simulink model "Sim_sixDOF"  (R2023a)
settings: Solver=ode4  StartTime=0.0  StopTime=100  FixedStep=0.1  RelTol=1e-3
values from neighbouring files (symbols this model uses):
  a0_s2 = 0    [computeAeroForces.m]
  a0_s3 = 0    [computeAeroForces.m]
  a0_s4 = 0.05    [computeAeroForces.m]
  a0_s5 = 0.05    [computeAeroForces.m]
  AR_s2 = b_s2/c_s2    [computeSurfacePos.m]
  AR_s3 = b_s3/c_s3    [computeSurfacePos.m]
  AR_s4 = (b_s4 + b_s5)/c_s4    [computeSurfacePos.m]
  AR_s5 = (b_s4 + b_s5)/c_s5    [computeSurfacePos.m]
  area_s2 = c_s2 * b_s2    [computeSurfacePos.m]
  area_s3 = c_s3 * b_s3    [computeSurfacePos.m]
  area_s4 = c_s4 * b_s4    [computeSurfacePos.m]
  area_s5 = c_s5 * b_s5    [computeSurfacePos.m]
  c_s2 = componentMassesAndGeom(3,2)    [computeSurfacePos.m]
  c_s3 = componentMassesAndGeom(4,2)    [computeSurfacePos.m]
  c_s4 = componentMassesAndGeom(1,2)    [computeSurfacePos.m]
  c_s5 = componentMassesAndGeom(2,2)    [computeSurfacePos.m]
  CD0_s2 = 0.01    [computeAeroForces.m]
  CD0_s3 = 0.01    [computeAeroForces.m]
  CD0_s4 = 0.01    [computeAeroForces.m]
  CD0_s5 = 0.01    [computeAeroForces.m]
  CDa_s2 = 1    [computeAeroForces.m]
  CDa_s3 = 1    [computeAeroForces.m]
  CDa_s4 = 1    [computeAeroForces.m]
  CDa_s5 = 1    [computeAeroForces.m]
  CL0_s2 = 0    [computeAeroForces.m]
  CL0_s3 = 0    [computeAeroForces.m]
  CL0_s4 = 0.05    [computeAeroForces.m]
  CL0_s5 = 0.05    [computeAeroForces.m]
  CM0_s2 = 0    [computeAeroForces.m]
  CM0_s3 = 0    [computeAeroForces.m]
  CM0_s4 = -0.05    [computeAeroForces.m]
  CM0_s5 = -0.05    [computeAeroForces.m]
  CMa_s2 = 0    [computeAeroForces.m]
  CMa_s3 = 0    [computeAeroForces.m]
  CMa_s4 = 0    [computeAeroForces.m]
  CMa_s5 = 0    [computeAeroForces.m]
  e_s2 = 0.8    [computeAeroForces.m]
  e_s3 = 0.8    [computeAeroForces.m]
  e_s4 = 0.9    [computeAeroForces.m]
  e_s5 = 0.9    [computeAeroForces.m]
  elevator_sA = 0.435    [Sim_sixDOFdriverScript.m]
  i_s2 = 0    [computeAeroForces.m]
  i_s3 = 0    [computeAeroForces.m]
  i_s4 = 0.05    [computeAeroForces.m]
  i_s5 = 0.05    [computeAeroForces.m]
  Jxx = 1    [Sim_sixDOFdriverScript.m]
  Jxy = 0.    (= 0)    [Sim_sixDOFdriverScript.m]
  Jxz = 3    [Sim_sixDOFdriverScript.m]
  Jyx = 2    [Sim_sixDOFdriverScript.m]
  Jyy = 2    [Sim_sixDOFdriverScript.m]
  Jyz = 0    [Sim_sixDOFdriverScript.m]
  Jzx = Jxz    (= 3)    [Sim_sixDOFdriverScript.m]
  Jzy = Jyz    (= 0)    [Sim_sixDOFdriverScript.m]
  Jzz = 2    [Sim_sixDOFdriverScript.m]
  leftaileron_sA = 0.192/2    (= 0.096)    [Sim_sixDOFdriverScript.m]
  LL = 0.8    [Sim_sixDOFdriverScript.m]
  mixMatrixInv = inv(mixMatrix)    [Sim_sixDOFdriverScript.m]
  MM = 0.8    [Sim_sixDOFdriverScript.m]
  n_s2 = [0; 0; -1]    [computeAeroForces.m]
  n_s3 = [0; 1; 0]    [computeAeroForces.m]
  n_s4 = [0; 0; -1]    [computeAeroForces.m]
  n_s5 = [0; 0; -1]    [computeAeroForces.m]
  NN = 0.8    [Sim_sixDOFdriverScript.m]
  rEarth = 6378100    [Sim_sixDOFdriverScript.m]
  rightaileron_sA = 0.192/2    (= 0.096)    [Sim_sixDOFdriverScript.m]
  ro = 1.225    [computeAeroForces.m]
  rudder_sA = 0.0333    [Sim_sixDOFdriverScript.m]
  totMass = sum(componentMassesAndGeom(:,1))    [computeMassProps.m]
  x_S2_B_B = (x_S2_B_B_nominal + [0.25*c_s2 0 0]') - x_cg    [computeMassProps.m]
  x_S3_B_B = (x_S3_B_B_nominal + [0.25*c_s3 0 0]') - x_cg    [computeMassProps.m]
  x_S4_B_B = (x_S4_B_B_nominal + [0.25*c_s4 0 0]') - x_cg    [computeMassProps.m]
  x_S5_B_B = (x_S5_B_B_nominal + [0.25*c_s5 0 0]') - x_cg    [computeMassProps.m]
libraries: aerolibutil x3, simulink_extras x3, matrix_library x2, sharedtransform x2, simulink x2, sharedutil x1, vrlib x1
(part 2 of 2)

== matlab function Sim_sixDOF/Equations of Motion/Aero Forces and Moments/F&M Right Wing and Servo Surface (S5)/F&M in Body/Force Due to Lift and Drag ==
  data: lift input; forceLiftDragS5_B output; drag input; v_B_A_B input; n_s5 input
function forceLiftDragS5_B = fcn(lift, drag, v_B_A_B, n_s5)

forceLiftDrag_w = lift*n_s5 - [drag; 0; 0];
alpha = atan2(v_B_A_B(3), v_B_A_B(1));
beta = asin(v_B_A_B(2) / norm(v_B_A_B));

c_S_B = [cos(alpha), 0, sin(alpha); 0, 1, 0; -sin(alpha), 0, cos(alpha)] ;
c_W_S = [cos(beta), sin(beta), 0; -sin(beta), cos(beta), 0; 0,0,1];
c_W_B = c_W_S * c_S_B;

forceLiftDragS5_B = c_W_B' * forceLiftDrag_w;

== matlab function Sim_sixDOF/Equations of Motion/Aero Forces and Moments/F&M Right Wing and Servo Surface (S5)/F&M in Body/Moment S5 ==
  data: momSurf input; momS5_B output; FliftdragS input; n_s5 input; x_S5_B_B input
function momS5_B = fcn(momSurf, FliftdragS, n_s5, x_S5_B_B)
% Compute the moment at the respective surface
crot = [0,0,0; 0,0,-1; 0,1,0];

momS5_B = momSurf * crot* n_s5 + (cross(x_S5_B_B, FliftdragS));

== matlab function Sim_sixDOF/Equations of Motion/TransKin_RotKin_TansDynam/Rotational Kinematics_Quaternions/NormalizeQuaternion ==
  data: qin input; qoutNorm output
function qoutNorm = NormalizeQuaternion(qin)
qinMag = norm(qin);
qoutNorm = qin/qinMag;

== matlab function Sim_sixDOF/Equations of Motion/Aero Forces and Moments/F&M Horiz Stab Surface (S2)/F&M in Body/Moment S2 ==
  data: momSurf input; momS2_B output; FliftdragS input; n_s2 input; x_S2_B_B input
function momS2_B = fcn(momSurf, FliftdragS, n_s2, x_S2_B_B)
% Compute the moment at the respective surface
crot = [0,0,0; 0,0,-1; 0,1,0];

momS2_B = momSurf * crot* n_s2 + (cross(x_S2_B_B, FliftdragS));

== matlab function Sim_sixDOF/Equations of Motion/TransKin_RotKin_TansDynam/Rotational Kinematics_Quaternions/quaternionMultiplication ==
  data: q1 input; qResult output; q2 input
function qResult = quaternionMultiplication(q1,q2)
q1imag = [q1(2); q1(3); q1(4)] ;
q2imag = [q2(2); q2(3); q2(4)];
qResultMag = q1(1)*q2(1) - dot(q1imag, q2imag);

qResultVect = q1(1)*q2imag + q2(1)*q1imag + cross(q1imag,q2imag);
qResult = [qResultMag; qResultVect];
end

== matlab function Sim_sixDOF/Equations of Motion/TransKin_RotKin_TansDynam/Rotational Kinematics_Quaternions/quaternionToeuler ==
  data: qin input; yaw_deg output; pitch_deg output; roll_deg output
function [yaw_deg, pitch_deg, roll_deg] = quaternionsToEulerZYX(qin)
% Function to transfrom quaternion to Euler Angles in Tait-Bryan yaw,
% pitch, roll angle sequence

roll = atan2(2*(qin(1)*qin(2) + qin(3)*qin(4)), 1-2*(qin(2)^2 + qin(3)^2));
temp1 = sqrt(1+2*(qin(1)*qin(3)-qin(2)*qin(4)));
temp2 = sqrt(1-2*(qin(1)*qin(3) - qin(2)*qin(4)));
pitch = -pi/2 + 2*atan2(temp1, temp2);
yaw = atan2(2*(qin(1)*qin(4) + qin(2)*qin(3)) ,1-2*(qin(3)^2 + qin(4)^2));

yaw_deg = rad2deg(yaw);
pitch_deg = rad2deg(pitch);
roll_deg = rad2deg(roll);

end

== matlab function Sim_sixDOF/Equations of Motion/Aero Forces and Moments/F&M Horiz Stab Surface (S3)/Compute Aero Lift and Drag ==
  data: alphaLocal output; v_B_A_B input; liftSurf output; dragSurf output; AR_s3 input; i_s3 input; n_s3 input; CL0_s3 input; CD0_s3 input; CDa_s3 input; a0_s3 input; e_s3 input; ro input; area_s3 input; rudderControl input; rudderarea_uControl input
function [alphaLocal, liftSurf, dragSurf] = fcn(v_B_A_B, AR_s3, i_s3, n_s3, CL0_s3, CD0_s3, CDa_s3, a0_s3, e_s3, ro, area_s3, rudderControl, rudderarea_uControl)
% Compute the lift and drag forces at the respective surface
% arSurf -> Aspect Ratio of respective surfaace
% ro -> air density (note: varies with altitude)
% v_infSurf -> total airspeed at the surface, i.e. Velocity of body w.r.t Inertial/ECEF as
% measured in body frame (|V_B_E_B|)
% v_B_A_B -> relative airspeed, where it is typically 
% v_B_E_B - c_B_N * v_A_N_N and v_A_N_N is the velocity of air mass w.r.t. NED 
% nSurf_B -> Normal force applied at surface
% eSurf -> Oswald efficiency
% alphaLocal0 -> Minimum drag Angle of Attack
delCLsPerdelMu = 3; % ~ About 3 per radian
v_infSurf = norm(v_B_A_B);
cSurfLocAlpha = 2*pi * (AR_s3/(2+AR_s3)); % Lift coefficient at the respective surface due to the local alpha (Angle of Attack)
alphaLocal = i_s3 - asin(dot(v_B_A_B,n_s3)/norm(v_B_A_B)); % in Radians
%cSurfLift = CL0_s3 + cSurfLocAlpha * alphaLocal; % Lift coefficient of surface
cSurfLift = CL0_s3 + cSurfLocAlpha * alphaLocal + (delCLsPerdelMu)*rudderControl*(rudderarea_uControl/area_s3); % Lift coefficient of surface
cSurfDrag = CD0_s3 + CDa_s3 *(alphaLocal - a0_s3)^2 + (cSurfLift^2/(pi*e_s3*AR_s3));

liftSurf = cSurfLift * 0.5 * ro * (v_infSurf^2)*area_s3;
dragSurf = cSurfDrag * 0.5 * ro * (v_infSurf^2)*area_s3;

== matlab function Sim_sixDOF/Equations of Motion/TransKin_RotKin_TansDynam/Translational Kinematics/cartesianTOgeodetic ==
  data: cartVecPos input; lat_deg output; lon_deg output; r output
function [lat_deg, lon_deg, r]= cartesionTOgeodetic(cartVecPos)
% Cartesion coordinates must be w.r.t. ECEF frame
rEarth = 6378100; %m
r = norm(cartVecPos);
lat_deg = asind(cartVecPos(3)/r);
lon_deg = atan2d(cartVecPos(2),cartVecPos(1));

== matlab function Sim_sixDOF/Equations of Motion/Aero Forces and Moments/F&M Horiz Stab Surface (S3)/Compute Aero Moment ==
  data: V_B_A_B input; momSurf output; alphaLocal input; CM0_s3 input; CMa_s3 input; ro input; area_s3 input; c_s3 input
function momSurf = fcn(V_B_A_B, alphaLocal, CM0_s3, CMa_s3, ro, area_s3, c_s3)
% Compute the Moment at the respective Surface
% v_infSurf -> total airspeed at the surface, i.e. Velocity of body w.r.t Inertial/ECEF as
% measured in body frame (|V_B_E_B|)
% ro -> air density (note: varies with altitude)
% chordSurf -> Chord of the surface area
% cSurfM0 -> Initial moment coefficient of surface
% cSurfMalpha -> Moment coefficient at the respective surface due to the
% local alpha (Angle of Attack)
v_infSurf = norm(V_B_A_B);
cSurfMom = CM0_s3 + CMa_s3*alphaLocal; % Moment coefficient of surface
momSurf = cSurfMom * 0.5 * ro * (v_infSurf^2)*area_s3 * c_s3;

== matlab function Sim_sixDOF/Equations of Motion/Aero Forces and Moments/F&M Horiz Stab Surface (S3)/F&M in Body/Force Due to Lift and Drag ==
  data: lift input; forceLiftDragS3_B output; drag input; v_B_A_B input; n_s3 input
function forceLiftDragS3_B = fcn(lift, drag, v_B_A_B, n_s3)

forceLiftDrag_w = lift*n_s3 - [drag; 0; 0];
alpha = atan2(v_B_A_B(3), v_B_A_B(1));
beta = asin(v_B_A_B(2) / norm(v_B_A_B));

c_S_B = [cos(alpha), 0, sin(alpha); 0, 1, 0; -sin(alpha), 0, cos(alpha)] ;
c_W_S = [cos(beta), sin(beta), 0; -sin(beta), cos(beta), 0; 0,0,1];
c_W_B = c_W_S * c_S_B;

forceLiftDragS3_B = c_W_B' * forceLiftDrag_w;

== matlab function Sim_sixDOF/Equations of Motion/Aero Forces and Moments/F&M Horiz Stab Surface (S3)/F&M in Body/Moment S3 ==
  data: momSurf input; momS3_B output; FliftdragS input; n_s3 input; x_S3_B_B input
function momS3_B = fcn(momSurf, FliftdragS, n_s3, x_S3_B_B)
% Compute the moment at the respective surface
crot = [0,0,0; 0,0,-1; 0,1,0];

momS3_B = momSurf * crot* n_s3 + (cross(x_S3_B_B, FliftdragS));

== matlab function Sim_sixDOF/Equations of Motion/TransKin_RotKin_TansDynam/Translational Kinematics/C_E_N ==
  data: lon_rad input; y output; lat_rad input
function y = NEDtoECEF(lon_rad, lat_rad)
% DCM to go from NED to ECEF frame

firstRot = [cos(lon_rad), cos(lon_rad), 0; -sin(lon_rad), cos(lon_rad), 0; 0, 0, 1;]; % Rotate about longitude first

secondRot = [0, 0, 1; 0, 1, 0; -1, 0,0]; % Left handed rotation of 90 deg 

thirdRot = [cos(lat_rad),0,sin(lat_rad); 0,1,0; -sin(lat_rad), 0, cos(lat_rad)];
% Multiply to get ECEF to NED DCM

c_NED_ECEF = thirdRot*secondRot*firstRot;
y = c_NED_ECEF';

== matlab function Sim_sixDOF/Equations of Motion/TransKin_RotKin_TansDynam/Rotational Kinematics_Euler/HinvMatrix ==
  data: pitchTheta input; hinv output; rollPhi input
function hinv = HinvMat(pitchTheta, rollPhi)
tThetasPhi = tan(pitchTheta) * sin(rollPhi);
tThetacPhi = tan(pitchTheta) * cos(rollPhi);
cPhi = cos(rollPhi);
sPhi = sin(rollPhi);
sPhiOvercTheta = sin(rollPhi)/cos(pitchTheta);
cPhiOvercTheta = cos(rollPhi)/cos(pitchTheta);

h = [1,tThetasPhi,tThetacPhi; 0,cPhi,-sPhi; 0,sPhiOvercTheta,cPhiOvercTheta];

hinv = h;

== matlab function Sim_sixDOF/Equations of Motion/Rotational Kinematics_Strapdown/Omega_B_N ==
  data: P_degPs input; y output; Q_degPs input; R_degPs input
function y = Omega_B_N(P_degPs,Q_degPs,R_degPs)
% Function used to generate cross product matrix of body rates (P,Q,R)
% w.r.t NED. This is basically a skew symmetric matrix
Omega_B_N = [0,-R_degPs,Q_degPs; R_degPs,0,-P_degPs; -Q_degPs,P_degPs,0];
y = Omega_B_N;

== matlab function Sim_sixDOF/Equations of Motion/Rotational Kinematics_Strapdown/dcmTOeuler ==
  data: inputDCM input; yaw_deg output; pitch_deg output; roll_deg output
function [yaw_deg, pitch_deg, roll_deg] = dcmTOEuler_TB(inputDCM)
% This function takes in a dcm and outputs the euler angles in a Tait-Bryan
% ZYX angle sequence
c12 = inputDCM(1,2);
c11 = inputDCM(1,1);
c13 = inputDCM(1,3);
c23 = inputDCM(2,3);
c33 = inputDCM(3,3);
yaw_deg = atand(c12/c11);
pitch_deg = -asind(c13);
roll_deg = atand(c23/c33);
end

== matlab function Sim_sixDOF/Equations of Motion/Rotational Kinematics_Quaternions/quaternionMultiplication ==
  data: q1 input; qResult output; q2 input
function qResult = quaternionMultiplication(q1,q2)
q1imag = [q1(2); q1(3); q1(4)] ;
q2imag = [q2(2); q2(3); q2(4)];
qResultMag = q1(1)*q2(1) - dot(q1imag, q2imag);

qResultVect = q1(1)*q2imag + q2(1)*q1imag + cross(q1imag,q2imag);
qResult = [qResultMag; qResultVect];
end

== matlab function Sim_sixDOF/Equations of Motion/Rotational Kinematics_Quaternions/quaternionToeuler ==
  data: qin input; yaw_deg output; pitch_deg output; roll_deg output
function [yaw_deg, pitch_deg, roll_deg] = quaternionsToEulerZYX(qin)
% Function to transfrom quaternion to Euler Angles in Tait-Bryan yaw,
% pitch, roll angle sequence

roll = atan2(2*(qin(1)*qin(2) + qin(3)*qin(4)), 1-2*(qin(2)^2 + qin(3)^2));
temp1 = sqrt(1+2*(qin(1)*qin(3)-qin(2)*qin(4)));
temp2 = sqrt(1-2*(qin(1)*qin(3) - qin(2)*qin(4)));
pitch = -pi/2 + 2*atan2(temp1, temp2);
yaw = atan2(2*(qin(1)*qin(4) + qin(2)*qin(3)) ,1-2*(qin(3)^2 + qin(4)^2));

yaw_deg = rad2deg(yaw);
pitch_deg = rad2deg(pitch);
roll_deg = rad2deg(roll);

end

== matlab function Sim_sixDOF/Equations of Motion/Rotational Kinematics_Quaternions/NormalizeQuaternion ==
  data: qin input; qoutNorm output
function qoutNorm = NormalizeQuaternion(qin)
qinMag = norm(qin);
qoutNorm = qin/qinMag;

== matlab function Sim_sixDOF/Equations of Motion/Rotational Dynamics/Using Cross Product Matrix/Omega Cross Matrix ==
  data: PQR input; omegaMat output
function omegaMat = fcn(PQR)
P = PQR(1); % deg
Q = PQR(2); % deg
R = PQR(3); % deg
omegaMat = [0 -R Q; R 0 -P; -Q P 0];
